simulink model "PSS2B_fmu"  (R2020a)
settings: Solver=VariableStepAuto  StartTime=0.0  StopTime=16.5  FixedStep=0.005  RelTol=1e-2
libraries: fmu_me_lib x2
settings Model: Creator=meagh  LastModifiedBy=meagh

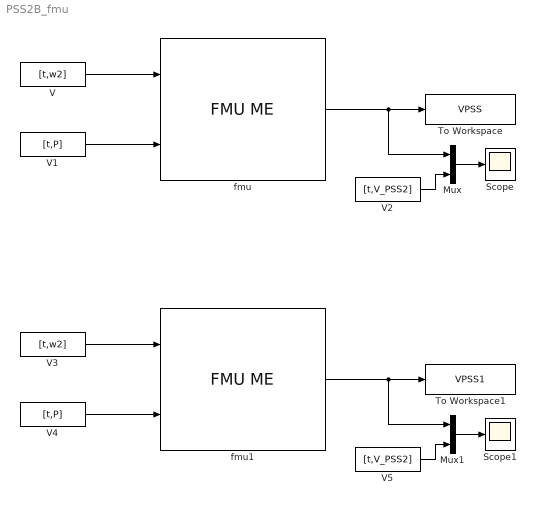
== system PSS2B_fmu ==
  Mux : Mux  Inputs=2
  Mux1 : Mux  Inputs=2
  Scope : Scope
  Scope1 : Scope
  To Workspace : ToWorkspace  VariableName=VPSS  SaveFormat=Timeseries  SampleTime=-1
  To Workspace1 : ToWorkspace  VariableName=VPSS1  SaveFormat=Timeseries  SampleTime=-1
  V : FromWorkspace  VariableName=[t,w2]
  V1 : FromWorkspace  VariableName=[t,P]
  V2 : FromWorkspace  VariableName=[t,V_PSS2]
  V3 : FromWorkspace  VariableName=[t,w2]
  V4 : FromWorkspace  VariableName=[t,P]
  V5 : FromWorkspace  VariableName=[t,V_PSS2]
  fmu : fmu_me_lib/FMU ME  Description=Simulates an FMU for Model Exchange 1.0 or Model Exchange 2.0.  dummy=0
  fmu1 : fmu_me_lib/FMU ME  Description=Simulates an FMU for Model Exchange 1.0 or Model Exchange 2.0.  dummy=0
  wires:
  V/1 -> fmu/1
  V1/1 -> fmu/2
  fmu/1 -> Mux/1, To Workspace/1
  Mux/1 -> Scope/1
  V2/1 -> Mux/2
  V3/1 -> fmu1/1
  V5/1 -> Mux1/2
  Mux1/1 -> Scope1/1
  V4/1 -> fmu1/2
  fmu1/1 -> Mux1/1, To Workspace1/1
